simulink model "untitled"  (R2023b)
settings: Solver=VariableStepAuto  StartTime=0.0  StopTime=10  RelTol=1e-3
settings Model: Creator=Wang  LastModifiedBy=Wang
settings DataIOCC: ExternalInput=[k, a]

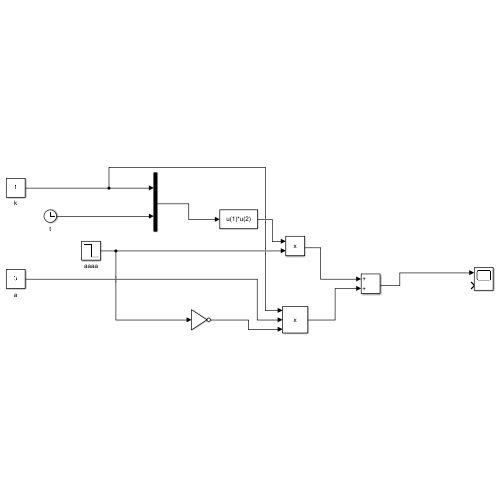
[thumbnail: Simulink's stored preview of the top-level diagram]
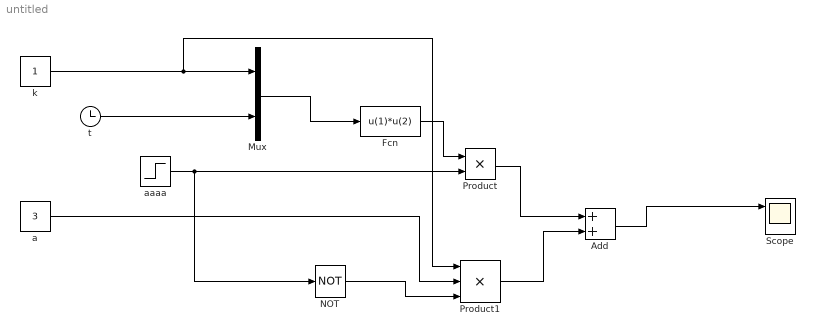
== system untitled ==
  Add : Sum
  Fcn : Fcn  Expr=u(1)*u(2)
  Mux : Mux  Inputs=2
  NOT : Logic  Operator=NOT  IconShape=distinctive  AllPortsSameDT=off  OutDataTypeStr=boolean
  Product : Product
  Product1 : Product  Inputs=3
  Scope : Scope  NumInputPorts=2
  a : Constant  Value=3
  aaaa : Step  Time=3  Before=1  After=0  SampleTime=0
  k : Constant
  t : Clock
  wires:
  Product/1 -> Add/1
  Product1/1 -> Add/2
  NOT/1 -> Product1/3
  Mux/1 -> Fcn/1
  Add/1 -> Scope/1
  Fcn/1 -> Product/1
  aaaa/1 -> NOT/1, Product/2
  t/1 -> Mux/2
  k/1 -> Product1/1, Mux/1
  a/1 -> Product1/2
